simulink model "robotdynamics"  (R2024b)
settings: Solver=VariableStepAuto  StartTime=0.0  StopTime=100  RelTol=1e-3
values from neighbouring files (symbols this model uses):
  g = 9.8    [untitled.m]
  initial_dtheta = [0; 0]    [untitled.m]
  initial_dtheta_d = inv(J) * cartesian_vel0    [untitled.m]
  initial_theta = [theta1_0; theta2_0]    [untitled.m]
  Kd = diag([40, 40])    [untitled.m]
  Kp = diag([100, 100])    [untitled.m]
  l1 = 1.0    (= 1)    [untitled.m]
  l2 = 1.0    (= 1)    [untitled.m]
  m1 = 1.0    (= 1)    [untitled.m]
  m2 = 1.0    (= 1)    [untitled.m]
settings Model: Creator=86195  LastModifiedBy=86195

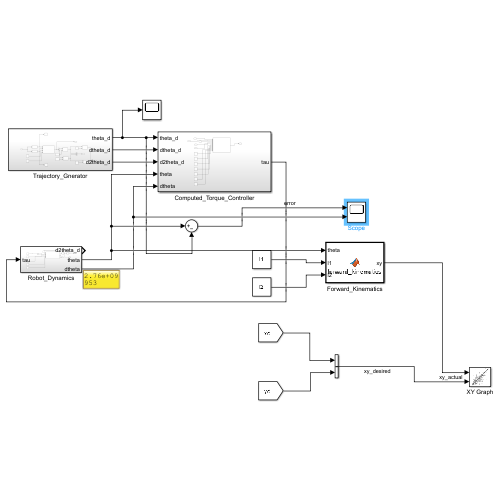
[thumbnail: Simulink's stored preview of the top-level diagram]
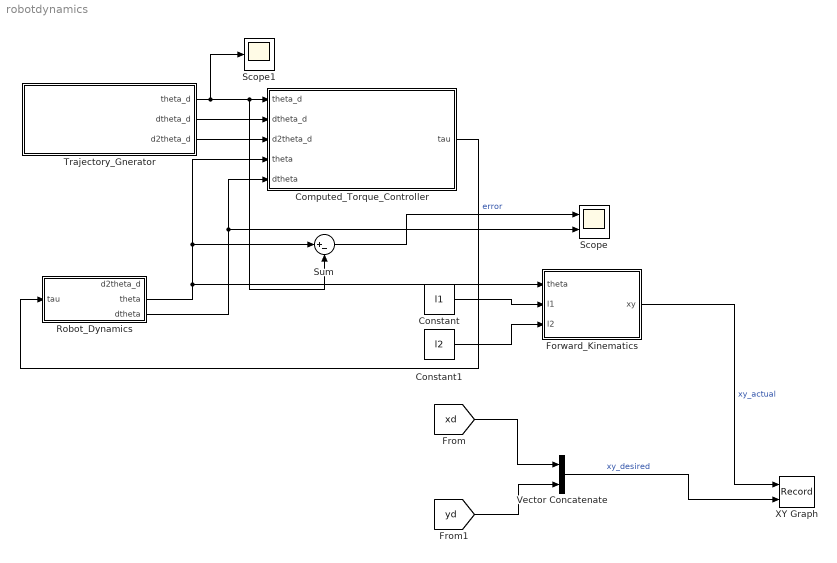
== system robotdynamics ==
  Computed_Torque_Controller : Subsystem
  Constant : Constant  Value=l1
  Constant1 : Constant  Value=l2
  Forward_Kinematics : MATLAB Function  TreatAsAtomicUnit=on
  Robot_Dynamics : Subsystem
  Scope : Scope  NumInputPorts=2
  Scope1 : Scope
  Sum : Sum  Inputs=|+-
  Trajectory_Gnerator : Subsystem
  Vector Concatenate : Concatenate
  XY Graph : Record  FileSettingsInternal="{\"entries\":[{\"content\":{\"excelSettings\":{\"content\":{},\"type\":\"Streamout.ExcelSettings\"}},\"type\":\"Streamout.FileSettingStorage\",\"uuid\":\"\"}],\"packageUris\":[\"http:\\/\\/schema.mathworks.com\\/mf0\\/streamout_blocks\\/R2020a\"],\"version\":\"1.0\"}"  Layout=[1 1]  SignalsInternal="{\"entries\":[{\"content\":{\"signals\":[{\"content\":{\"blockPath\":[],\"dimensions\":[2,1],\"domain\":\"\",\"hasChildren\":true,\"lineColor\":\"#fe330a\",\"lineWidth\":2,\"port\":1,\"sid\":[\"\"],\"signalID\":1,\"signalName\":\"xy_actual\"},\"type\":\"RecordBlkView.Signal\",\"uuid\":\"\"},{\"content\":{\"blockPath\":[],\"channel\":[1,1],\"dimensions\":[2,1],\"domain\":\"\",\"lineColor\":\"#d95319\",\"lineWidth\":2,\"parentID\":1,\"plots\":[ 1 ],\"port\":1,\"sid\":[\"\"],\"signalID\":2,\"signalName\":\"xy_actual\"},\"type\":\"RecordBlkView.Signal\",\"uuid\":\"\"},{\"content\":{\"blockPath\":[],\"dimensions\":[2],\"domain\":\"\",\"hasChildren\":true,\"lineColor\":\"#0072bd\",\"lineWidth\":2,\"port\":2,\"sid\":[\"\"],\"signalID\":3,\"signalName\":\"xy_desired\"},\"type\":\"RecordBlkView.Signal\",\"uuid\":\"\"},{\"content\":{\"blockPath\":[],\"channel\":[1],\"dimensions\":[2],\"domain\":\"\",\"lineColor\":\"#7e2f8e\",\"lineWidth\":2,\"parentID\":3,\"plots\":[ 1 ],\"port\":2,\"sid\":[\"\"],\"signalID\":4,\"signalName\":\"xy_desired\"},\"type\":\"RecordBlkView.Signal\",\"uuid\":\"\"},{\"content\":{\"blockPath\":[],\"channel\":[2,1],\"dimensions\":[2,1],\"domain\":\"\",\"lineColor\":\"#77ac30\",\"lineWidth\":2,\"parentID\":1,\"plots\":[ 1 ],\"port\":1,\"sid\":[\"\"],\"signalID\":5,\"signalName\":\"xy_actual\"},\"type\":\"RecordBlkView.Signal\",\"uuid\":\"\"},{\"content\":{\"blockPath\":[],\"channel\":[2],\"dimensions\":[2],\"domain\":\"\",\"lineColor\":\"#4dbeee\",\"lineWidth\":2,\"parentID\":3,\"plots\":[ 1 ],\"port\":2,\"sid\":[\"\"],\"signalID\":6,\"signalName\":\"xy_desired\"},\"type\":\"RecordBlkView.Signal\",\"uuid\":\"\"}]},\"type\":\"RecordBlkView.InputSignals\",\"uuid\":\"\"}],\"packageUris\":[\"http:\\/\\/schema.mathworks.com\\/mf0\\/streamout_blocks\\/R2020a\"],\"version\":\"1.0\"}"  VisualizationBindings="{\"xyplotplugin\":{\"info\":[{\"series\":[{\"bindingParametersList\":[{\"parameter\":\"X-Axis\",\"signalID\":4,\"signalName\":\"xy_desired(1)\"},{\"parameter\":\"Y-Axis\",\"signalID\":6,\"signalName\":\"xy_desired(2)\"},{\"parameter\":\"X-Axis\",\"signalID\":4,\"signalName\":\"xy_desired(1)\"},{\"parameter\":\"Y-Axis\",\"signalID\":6,\"signalName\":\"xy_desired(2)\"}],\"seriesID\":0},{\"bindingParametersList\":[{\"parameter\":\"X-Axis\",\"signalID\":2,\"signalName\":\"xy_actual(1,1)\"},{\"parameter\":\"Y-Axis\",\"signalID\":5,\"signalName\":\"xy_actual(2,1)\"}],\"seriesID\":1}],\"subplotID\":1}]}}"  CompatibilityTag=XY
  wires:
  Trajectory_Gnerator/1(theta_d) -> Scope1/1, Sum/2, Computed_Torque_Controller/1(theta_d)
  Trajectory_Gnerator/2(dtheta_d) -> Computed_Torque_Controller/2(dtheta_d)
  Trajectory_Gnerator/3(d2theta_d) -> Computed_Torque_Controller/3(d2theta_d)
  Robot_Dynamics/2(theta) -> Computed_Torque_Controller/4(theta), Sum/1, Forward_Kinematics/1(theta)
  Robot_Dynamics/3(dtheta) -> Computed_Torque_Controller/5(dtheta), Scope/2
  Computed_Torque_Controller/1(tau) -> Robot_Dynamics/1(tau)
  Sum/1 -> Scope/1  "error"
  [xd] -> Vector Concatenate/1
  [yd] -> Vector Concatenate/2
  Vector Concatenate/1 -> XY Graph/2  "xy_desired"
  Forward_Kinematics/1(xy) -> XY Graph/1  "xy_actual"
  Constant/1 -> Forward_Kinematics/2(l1)
  Constant1/1 -> Forward_Kinematics/3(l2)

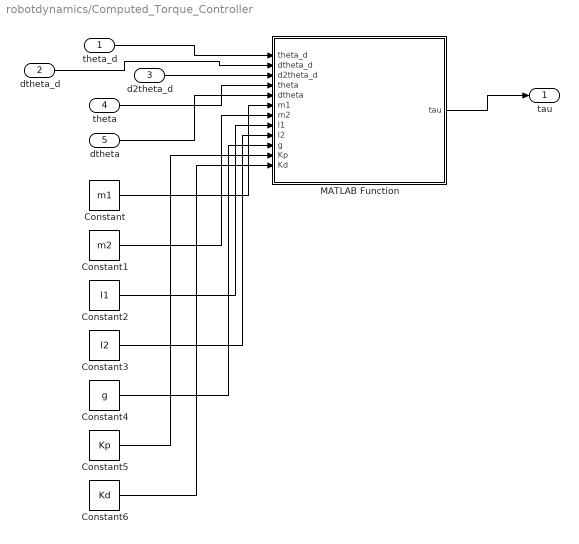
== system robotdynamics/Computed_Torque_Controller ==
  theta_d : Inport
  dtheta_d : Inport  Port=2
  d2theta_d : Inport  Port=3
  theta : Inport  Port=4
  dtheta : Inport  Port=5
  Constant : Constant  Value=m1
  Constant1 : Constant  Value=m2
  Constant2 : Constant  Value=l1
  Constant3 : Constant  Value=l2
  Constant4 : Constant  Value=g
  Constant5 : Constant  Value=Kp
  Constant6 : Constant  Value=Kd
  MATLAB Function : MATLAB Function  TreatAsAtomicUnit=on
  tau : Outport
  wires:
  theta_d/1 -> MATLAB Function/1(theta_d)
  dtheta_d/1 -> MATLAB Function/2(dtheta_d)
  theta/1 -> MATLAB Function/4(theta)
  dtheta/1 -> MATLAB Function/5(dtheta)
  MATLAB Function/1(tau) -> tau/1
  Constant/1 -> MATLAB Function/6(m1)
  Constant1/1 -> MATLAB Function/7(m2)
  Constant3/1 -> MATLAB Function/9(l2)
  Constant2/1 -> MATLAB Function/8(l1)
  Constant4/1 -> MATLAB Function/10(g)
  Constant5/1 -> MATLAB Function/11(Kp)
  Constant6/1 -> MATLAB Function/12(Kd)
  d2theta_d/1 -> MATLAB Function/3(d2theta_d)

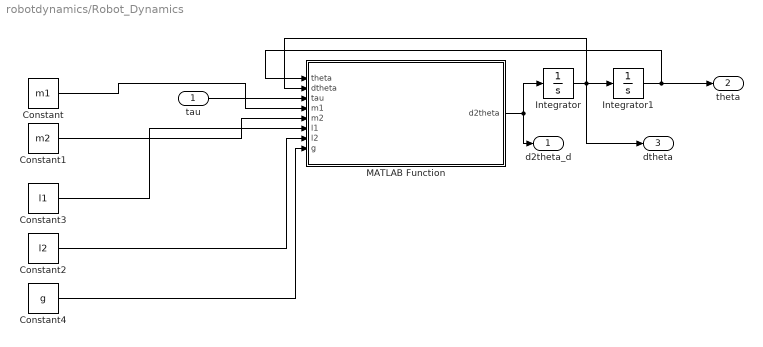
== system robotdynamics/Robot_Dynamics ==
  tau : Inport
  Constant : Constant  Value=m1
  Constant1 : Constant  Value=m2
  Constant2 : Constant  Value=l2
  Constant3 : Constant  Value=l1
  Constant4 : Constant  Value=g
  Integrator : Integrator  InitialCondition=initial_dtheta
  Integrator1 : Integrator  InitialCondition=initial_theta
  MATLAB Function : MATLAB Function  TreatAsAtomicUnit=on
  d2theta_d : Outport
  theta : Outport  Port=2
  dtheta : Outport  Port=3
  wires:
  MATLAB Function/1(d2theta) -> d2theta_d/1, Integrator/1
  Integrator/1 -> MATLAB Function/2(dtheta), dtheta/1, Integrator1/1
  Integrator1/1 -> MATLAB Function/1(theta), theta/1
  tau/1 -> MATLAB Function/3(tau)
  Constant/1 -> MATLAB Function/4(m1)
  Constant1/1 -> MATLAB Function/5(m2)
  Constant3/1 -> MATLAB Function/6(l1)
  Constant2/1 -> MATLAB Function/7(l2)
  Constant4/1 -> MATLAB Function/8(g)

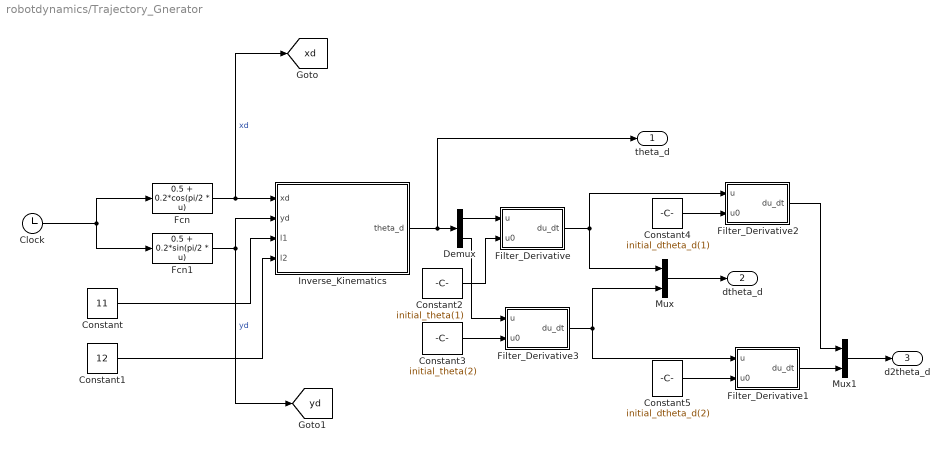
== system robotdynamics/Trajectory_Gnerator ==
  Clock : Clock
  Constant : Constant  Value=11
  Constant1 : Constant  Value=12
  Constant2 : Constant  Value=initial_theta(1)
  Constant3 : Constant  Value=initial_theta(2)
  Constant4 : Constant  Value=initial_dtheta_d(1)
  Constant5 : Constant  Value=initial_dtheta_d(2)
  Demux : Demux  Outputs=2
  Fcn : Fcn  Expr=0.5 + 0.2*cos(pi/2 * u)
  Fcn1 : Fcn  Expr=0.5 + 0.2*sin(pi/2 * u)
  Filter_Derivative : Subsystem
  Filter_Derivative1 : Subsystem
  Filter_Derivative2 : Subsystem
  Filter_Derivative3 : Subsystem
  Inverse_Kinematics : MATLAB Function  TreatAsAtomicUnit=on
  Mux : Mux  Inputs=2
  Mux1 : Mux  Inputs=2
  theta_d : Outport
  dtheta_d : Outport  Port=2
  d2theta_d : Outport  Port=3
  tag scope: xd=global, yd=global
  wires:
  Fcn/1 -> [xd], Inverse_Kinematics/1(xd)  "xd"
  Fcn1/1 -> [yd], Inverse_Kinematics/2(yd)  "yd"
  Constant/1 -> Inverse_Kinematics/3(l1)
  Constant1/1 -> Inverse_Kinematics/4(l2)
  Clock/1 -> Fcn/1, Fcn1/1
  Filter_Derivative/1(du_dt) -> Mux/1, Filter_Derivative2/1(u)
  Inverse_Kinematics/1(theta_d) -> Demux/1, theta_d/1
  Demux/1 -> Filter_Derivative/1(u)
  Constant2/1 -> Filter_Derivative/2(u0)
  Demux/2 -> Filter_Derivative3/1(u)
  Constant3/1 -> Filter_Derivative3/2(u0)
  Constant4/1 -> Filter_Derivative2/2(u0)
  Filter_Derivative3/1(du_dt) -> Filter_Derivative1/1(u), Mux/2
  Constant5/1 -> Filter_Derivative1/2(u0)
  Mux/1 -> dtheta_d/1
  Filter_Derivative2/1(du_dt) -> Mux1/1
  Filter_Derivative1/1(du_dt) -> Mux1/2
  Mux1/1 -> d2theta_d/1

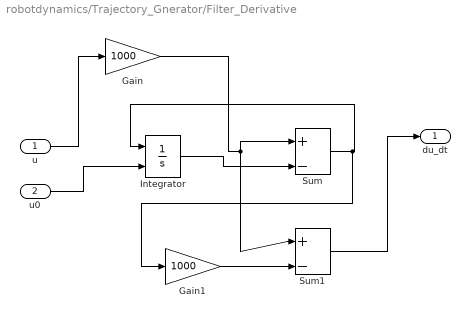
== system robotdynamics/Trajectory_Gnerator/Filter_Derivative ==
  u : Inport
  u0 : Inport  Port=2
  Gain : Gain  Gain=1000
  Gain1 : Gain  Gain=1000
  Integrator : Integrator  InitialConditionSource=external
  Sum : Sum  Inputs=|+-
  Sum1 : Sum  Inputs=|+-
  du_dt : Outport
  wires:
  u0/1 -> Integrator/2
  u/1 -> Gain/1
  Gain/1 -> Sum1/1, Sum/1
  Integrator/1 -> Sum/2
  Sum/1 -> Gain1/1, Integrator/1
  Gain1/1 -> Sum1/2
  Sum1/1 -> du_dt/1

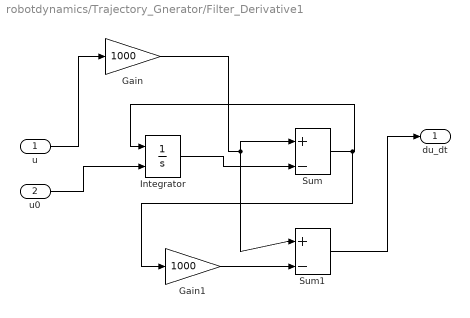
== system robotdynamics/Trajectory_Gnerator/Filter_Derivative1 ==
  u : Inport
  u0 : Inport  Port=2
  Gain : Gain  Gain=1000
  Gain1 : Gain  Gain=1000
  Integrator : Integrator  InitialConditionSource=external
  Sum : Sum  Inputs=|+-
  Sum1 : Sum  Inputs=|+-
  du_dt : Outport
  wires:
  u0/1 -> Integrator/2
  u/1 -> Gain/1
  Gain/1 -> Sum1/1, Sum/1
  Integrator/1 -> Sum/2
  Sum/1 -> Gain1/1, Integrator/1
  Gain1/1 -> Sum1/2
  Sum1/1 -> du_dt/1

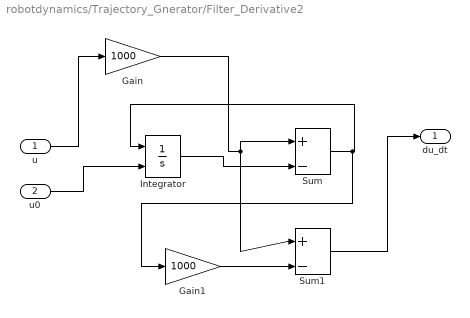
== system robotdynamics/Trajectory_Gnerator/Filter_Derivative2 ==
  u : Inport
  u0 : Inport  Port=2
  Gain : Gain  Gain=1000
  Gain1 : Gain  Gain=1000
  Integrator : Integrator  InitialConditionSource=external
  Sum : Sum  Inputs=|+-
  Sum1 : Sum  Inputs=|+-
  du_dt : Outport
  wires:
  u0/1 -> Integrator/2
  u/1 -> Gain/1
  Gain/1 -> Sum1/1, Sum/1
  Integrator/1 -> Sum/2
  Sum/1 -> Gain1/1, Integrator/1
  Gain1/1 -> Sum1/2
  Sum1/1 -> du_dt/1

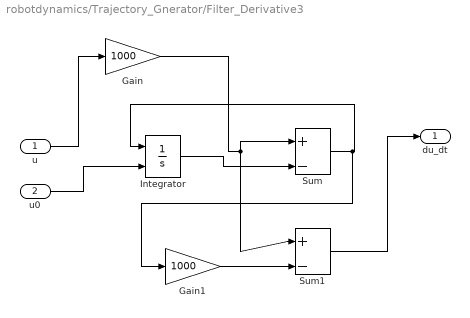
== system robotdynamics/Trajectory_Gnerator/Filter_Derivative3 ==
  u : Inport
  u0 : Inport  Port=2
  Gain : Gain  Gain=1000
  Gain1 : Gain  Gain=1000
  Integrator : Integrator  InitialConditionSource=external
  Sum : Sum  Inputs=|+-
  Sum1 : Sum  Inputs=|+-
  du_dt : Outport
  wires:
  u0/1 -> Integrator/2
  u/1 -> Gain/1
  Gain/1 -> Sum1/1, Sum/1
  Integrator/1 -> Sum/2
  Sum/1 -> Gain1/1, Integrator/1
  Gain1/1 -> Sum1/2
  Sum1/1 -> du_dt/1

== matlab function robotdynamics/Computed_Torque_Controller/MATLAB Function ==
  data: theta_d input; tau output; dtheta_d input; d2theta_d input; theta input; dtheta input; m1 input; m2 input; l1 input; l2 input; g input; Kp input; Kd input
function tau = computed_torque_law(theta_d, dtheta_d, d2theta_d, theta, dtheta, m1, m2, l1, l2, g, Kp, Kd)
%#codegen
% ===================================================================
%  完整版计算力矩控制器 (理论性能好，但对模型敏感，容易不稳定)
% ===================================================================

% --- 1. 计算误差 ---
e = theta_d - theta;   % 位置误差
de = dtheta_d - dtheta; % 速度误差

% --- 2. 计算外环PD控制输入 u ---
% u 是一个期望的“线性系统”加速度
u = d2theta_d + Kp*e + Kd*de;

% --- 3. 建立控制器内部的动力学模型估计 M_hat, C_hat, G_hat ---
% 这部分代码必须与 Robot_Dynamics 中的完全一致
lc1 = l1 / 2;
lc2 = l2 / 2;
th1 = theta(1);
th2 = theta(2);
dth1 = dtheta(1);
dth2 = dtheta(2);

% 惯量矩阵 M_hat(theta)
m11 = m1*lc1^2 + m2*(l1^2 + lc2^2 + 2*l1*lc2*cos(th2));
m12 = m2*(lc2^2 + l1*lc2*cos(th2));
m21 = m12;
m22 = m2*lc2^2;
M_hat = [m11, m12; m21, m22];

% 科里奥利/向心力矩阵 C_hat(theta, dtheta)
c11 = -m2*l1*lc2*sin(th2)*dth2;
c12 = -m2*l1*lc2*sin(th2)*(dth1 + dth2);
c21 = m2*l1*lc2*sin(th2)*dth1;
c22 = 0;
C_hat = [c11, c12; c21, c22];

% 重力项 G_hat(theta)
g1 = (m1*lc1 + m2*l1)*g*cos(th1) + m2*lc2*g*cos(th1 + th2);
g2 = m2*lc2*g*cos(th1 + th2);
G_hat = [g1; g2];

% --- 4. 计算最终力矩 tau ---
% 公式为： tau = M_hat*u + C_hat*dtheta + G_hat
tau = M_hat*u + C_hat*dtheta + G_hat;

== matlab function robotdynamics/Robot_Dynamics/MATLAB Function ==
  data: theta input; d2theta output; dtheta input; tau input; m1 input; m2 input; l1 input; l2 input; g input
% 将所有物理参数作为输入
function d2theta = robot_dynamics_eq(theta, dtheta, tau, m1, m2, l1, l2, g)
%#codegen

% ---- 不再需要evalin ----

% 为了简化，假设质心在中心
lc1 = l1 / 2;
lc2 = l2 / 2;

th1 = theta(1);
th2 = theta(2);
dth1 = dtheta(1);
dth2 = dtheta(2);

% ... 后面计算 M, C, G 的代码保持不变 ...
% 惯量矩阵 M(theta)
m11 = m1*lc1^2 + m2*(l1^2 + lc2^2 + 2*l1*lc2*cos(th2));
m12 = m2*(lc2^2 + l1*lc2*cos(th2));
m21 = m12;
m22 = m2*lc2^2;
M = [m11, m12; m21, m22];

% 科里奥利/向心力矩阵 C(theta, dtheta)
c11 = -m2*l1*lc2*sin(th2)*dth2;
c12 = -m2*l1*lc2*sin(th2)*(dth1 + dth2);
c21 = m2*l1*lc2*sin(th2)*dth1;
c22 = 0;
C = [c11, c12; c21, c22];

% 重力项 G(theta)
g1 = (m1*lc1 + m2*l1)*g*cos(th1) + m2*lc2*g*cos(th1 + th2);
g2 = m2*lc2*g*cos(th1 + th2);
G = [g1; g2];

% ... 前面的代码不变 ...

% 计算角加速度 (修改前)
% d2theta = inv(M) * (tau - C*dtheta - G);
% d2theta = M \ (tau - C*dtheta - G); % M\rhs 优于 inv(M)*rhs

% 计算角加速度 (修改后，增加阻尼)
delta = 1e-6; % 定义一个很小的阻尼值
d2theta = (M + eye(2)*delta) \ (tau - C*dtheta - G);

== matlab function robotdynamics/Trajectory_Gnerator/Inverse_Kinematics ==
  data: xd input; theta_d output; yd input; l1 input; l2 input
function theta_d = inverse_kinematics(xd, yd, l1, l2)
%#codegen
% This function calculates the inverse kinematics for a 2-DOF planar arm.

% Calculate theta2
% Ensure the value inside acos is within the valid range [-1, 1] to avoid numerical errors.
val = (xd^2 + yd^2 - l1^2 - l2^2) / (2 * l1 * l2);
if val > 1.0
    val = 1.0;
elseif val < -1.0
    val = -1.0;
end

% We choose the "elbow up" solution, which is common in robotics.
% Using atan2 for a more robust calculation of the angle from its cosine.
theta2 = atan2(-sqrt(1 - val^2), val); 

% Calculate theta1
k1 = l1 + l2 * cos(theta2);
k2 = l2 * sin(theta2);
theta1 = atan2(yd, xd) - atan2(k2, k1);

theta_d = [theta1; theta2];

== matlab function robotdynamics/Forward_Kinematics ==
  data: theta input; xy output; l1 input; l2 input
% 将l1, l2作为函数输入
function xy = forward_kinematics(theta, l1, l2)
%#codegen

% ---- 不再需要evalin ----
% l1 = evalin('base', 'l1');
% l2 = evalin('base', 'l2');

x = l1*cos(theta(1)) + l2*cos(theta(1)+theta(2));
y = l1*sin(theta(1)) + l2*sin(theta(1)+theta(2));
xy = [x; y];
